simulink library "link_subsystem_lib_test"  (Simulink 8.4)
settings: Solver=ode45  StartTime=0.0  StopTime=10.0  RelTol=1e-3
settings Model: Creator=arnaud  LastModifiedBy=arnaud

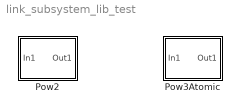
== system link_subsystem_lib_test ==
  Pow2 : Subsystem
  Pow3Atomic : Subsystem  TreatAsAtomicUnit=on

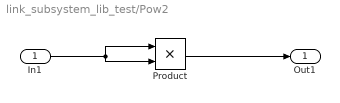
== system link_subsystem_lib_test/Pow2 ==
  In1 : Inport  PortDimensions=1  SampleTime=0
  Product : Product
  Out1 : Outport  PortDimensions=1  SampleTime=0
  wires:
  In1/1 -> Product/2, Product/1
  Product/1 -> Out1/1

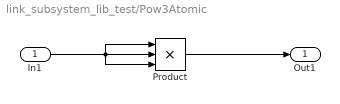
== system link_subsystem_lib_test/Pow3Atomic ==
  In1 : Inport  PortDimensions=1  SampleTime=0
  Product : Product  Inputs=3
  Out1 : Outport  PortDimensions=1  SampleTime=0
  wires:
  Product/1 -> Out1/1
  In1/1 -> Product/3, Product/2, Product/1
